simulink model "active_suspension_sim"  (Simulink 9.1)
settings: Solver=ode45  StartTime=0.0  StopTime=5  RelTol=1e-3
values from neighbouring files (symbols this model uses):
  A = [[0 1 0 0 0];[-(cw+cs)/mw -ds/mw cs/mw ds/mw -1/mw];[0 0 0 1 0];[cs/mc ds/mc -cs/mc -ds/mc 1/mc];[0 0 0 0 -1/tau]]    [active_suspension_ctrl_design.m]
  B1 = [B H]    [active_suspension_ctrl_design.m]
  C = [[-1 0 1 0 0];[cs/mc ds/mc -cs/mc -ds/mc 1/mc]]    [active_suspension_ctrl_design.m]
  C1 = eye(5)    [active_suspension_ctrl_design.m]
  D1 = zeros(5,2)    [active_suspension_ctrl_design.m]
  ds = 2200    [active_suspension_ctrl_design.m]
undefined symbols (not defined in the file or in its folder): K
libraries: simulink x3
settings Model: Creator=JonasMac  LastModifiedBy=joses
settings DataIOCC: LimitDataPoints=on  SignalLoggingSaveFormat=ModelDataLogs
settings OptimizationCC: BlockReduction=off  BooleanDataType=off
settings DebuggingCC: SaveWithParameterizedLinksMsg=none  SignalResolutionControl=TryResolveAllWithWarning  MultiTaskDSMMsg=warning  MultiTaskCondExecSysMsg=none
settings HardwareCC: TargetUnknown=on
settings GRTTargetCC: CombineOutputUpdateFcns=on  GRTInterface=off

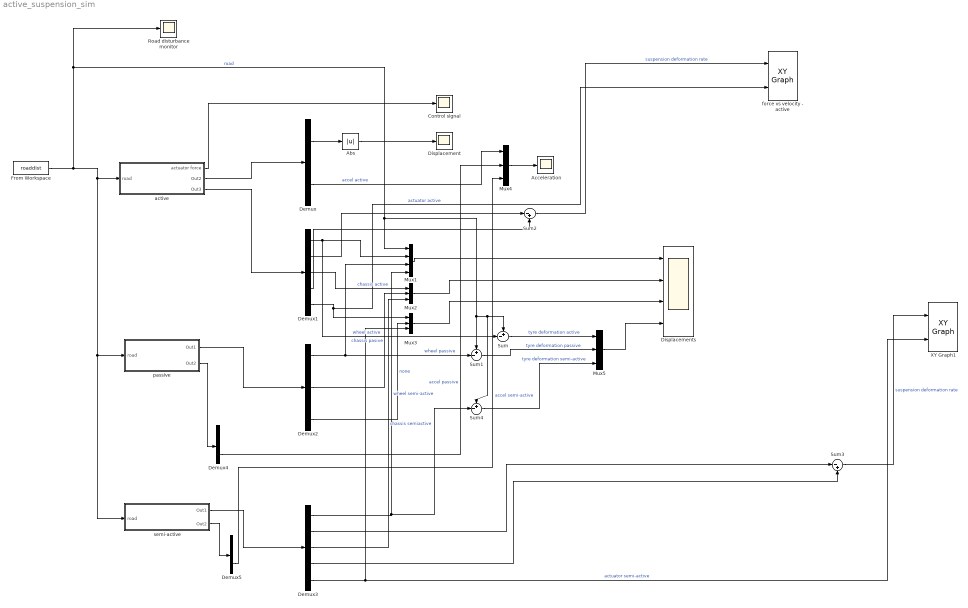
== system active_suspension_sim ==
  Abs : Abs
  Acceleration : Scope
  Control signal : Scope
  Demux : Demux  Outputs=2
  Demux1 : Demux  Outputs=5
  Demux2 : Demux  Outputs=5
  Demux3 : Demux  Outputs=5
  Demux4 : Demux  Outputs=2
  Demux5 : Demux  Outputs=2
  Displacement : Scope
  Displacements : Scope  NumInputPorts=4
  From Workspace : FromWorkspace  VariableName=roaddist  SampleTime=0
  Mux1 : Mux
  Mux{2..5} (4 alike) : Mux  Inputs=3
  Road disturbance monitor : Scope
  Sum : Sum  Inputs=+-|
  Sum1 : Sum  Inputs=+-|
  Sum2 : Sum  Inputs=|-+
  Sum3 : Sum  Inputs=|-+
  Sum4 : Sum  Inputs=+-|
  XY Graph1 : simulink/Sinks/XY Graph  xmin=-inf  xmax=inf  ymin=-inf  ymax=inf  st=.01
  active : Subsystem
  force vs velocity - active : simulink/Sinks/XY Graph  xmin=-inf  xmax=inf  ymin=-inf  ymax=inf  st=.01
  passive : Subsystem
  semi-active : Subsystem
  wires:
  Demux/1 -> Abs/1
  Abs/1 -> Displacement/1
  Mux1/1 -> Displacements/1
  Mux2/1 -> Displacements/2
  Mux3/1 -> Displacements/3
  Demux1/1 -> Sum/2, Mux1/2  "wheel active"
  Demux2/1 -> Sum1/2, Mux1/3  "wheel passive"
  Demux1/3 -> Mux2/1  "chassis active"
  Demux2/3 -> Mux2/2  "chassis pasive"
  Demux1/5 -> force vs velocity - active/2, Mux3/1  "actuator active"
  Demux2/5 -> Mux3/2  "none"
  Mux5/1 -> Displacements/4
  Sum/1 -> Mux5/1  "tyre deformation active"
  Sum1/1 -> Mux5/2  "tyre deformation passive"
  Demux1/2 -> Sum2/1
  Demux1/4 -> Sum2/2
  Sum2/1 -> force vs velocity - active/1  "suspension deformation rate"
  From Workspace/1 -> Road disturbance monitor/1, Sum1/1, Sum4/1, Sum/1, Mux1/1, semi-active/1(road), passive/1(road), active/1(road)  "road"
  active/1(actuator force) -> Control signal/1
  active/2(Out2) -> Demux/1
  active/3(Out3) -> Demux1/1
  passive/1(Out1) -> Demux2/1
  semi-active/1(Out1) -> Demux3/1
  Demux3/1 -> Sum4/2, Mux1/4  "wheel semi-active"
  Demux3/3 -> Mux2/3  "chassis semiactive"
  Demux3/5 -> XY Graph1/2, Mux3/3  "actuator semi-active"
  Sum3/1 -> XY Graph1/1  "suspension deformation rate"
  Demux3/4 -> Sum3/2
  Demux3/2 -> Sum3/1
  Sum4/1 -> Mux5/3  "tyre deformation semi-active"
  Mux4/1 -> Acceleration/1
  Demux/2 -> Mux4/1  "accel active"
  semi-active/2(Out2) -> Demux5/1
  Demux5/2 -> Mux4/3  "accel semi-active"
  passive/2(Out2) -> Demux4/1
  Demux4/2 -> Mux4/2  "accel passive"

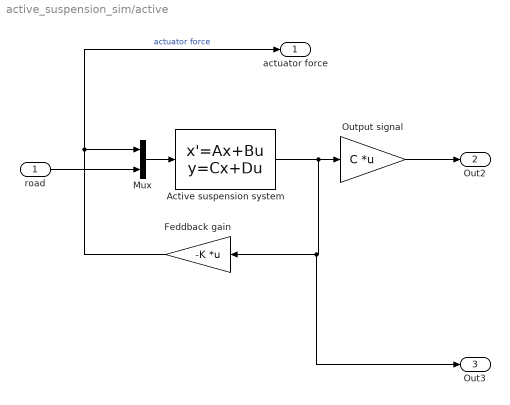
== system active_suspension_sim/active ==
  road : Inport
  Active suspension system : StateSpace  A=A  B=B1  C=C1  D=D1
  Feddback gain : Gain  Gain=-K  Multiplication=Matrix(K*u)
  Mux : Mux  Inputs=2
  Output signal : Gain  Gain=C  Multiplication=Matrix(K*u)
  actuator force : Outport
  Out2 : Outport  Port=2
  Out3 : Outport  Port=3
  wires:
  Active suspension system/1 -> Out3/1, Feddback gain/1, Output signal/1
  Feddback gain/1 -> actuator force/1, Mux/1  "actuator force"
  Mux/1 -> Active suspension system/1
  road/1 -> Mux/2
  Output signal/1 -> Out2/1

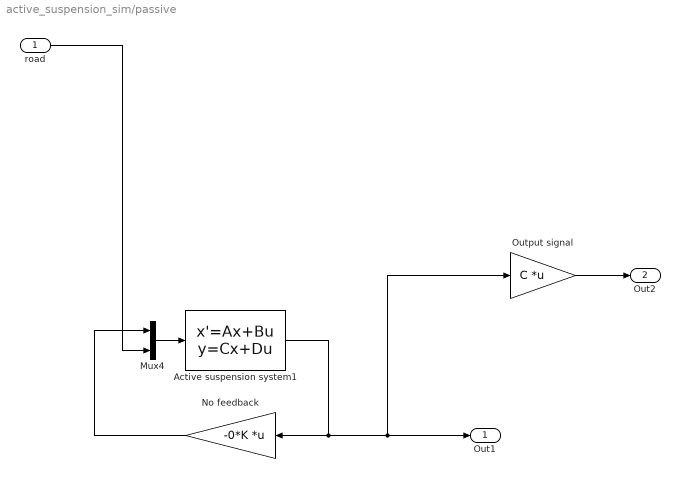
== system active_suspension_sim/passive ==
  road : Inport
  Active suspension system1 : StateSpace  A=A  B=B1  C=C1  D=D1
  Mux4 : Mux  Inputs=2
  No feedback : Gain  Gain=-0*K  Multiplication=Matrix(K*u)
  Output signal : Gain  Gain=C  Multiplication=Matrix(K*u)
  Out1 : Outport
  Out2 : Outport  Port=2
  wires:
  road/1 -> Mux4/2
  Active suspension system1/1 -> Output signal/1, Out1/1, No feedback/1
  Mux4/1 -> Active suspension system1/1
  No feedback/1 -> Mux4/1
  Output signal/1 -> Out2/1

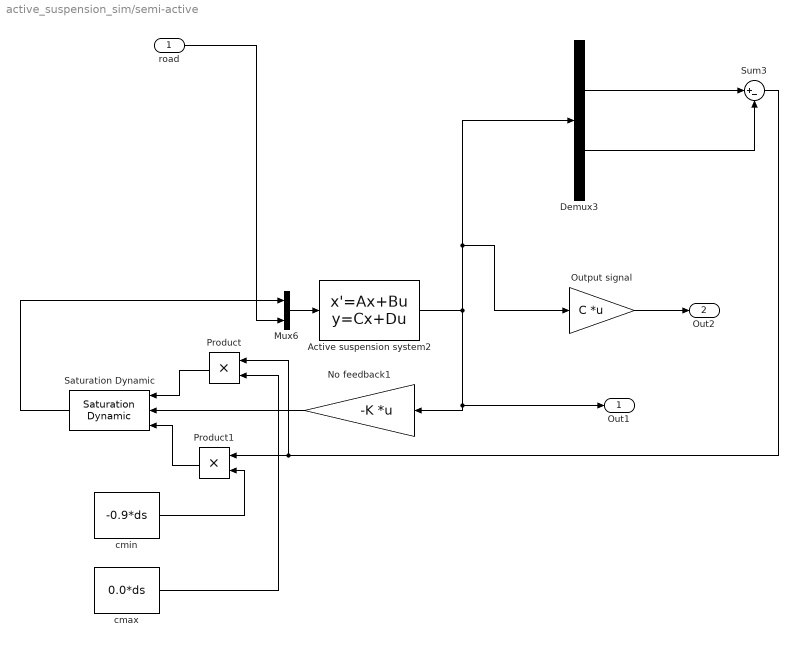
== system active_suspension_sim/semi-active ==
  road : Inport
  Active suspension system2 : StateSpace  A=A  B=B1  C=C1  D=D1
  Demux3 : Demux  Outputs=5
  Mux6 : Mux  Inputs=2
  No feedback1 : Gain  Gain=-K  Multiplication=Matrix(K*u)
  Output signal : Gain  Gain=C  Multiplication=Matrix(K*u)
  Product : Product
  Product1 : Product
  Saturation Dynamic : simulink/Discontinuities/Saturation Dynamic  OutMin=[]  OutMax=[]  OutDataTypeStr=Inherit: Same as second input  OutDataType=fixdt(1, 16)  OutScaling=2^-10  DoSatur=off
  Sum3 : Sum  Inputs=|+-
  cmax : Constant  Value=0.0*ds
  cmin : Constant  Value=-0.9*ds
  Out1 : Outport
  Out2 : Outport  Port=2
  wires:
  Active suspension system2/1 -> Output signal/1, Demux3/1, Out1/1, No feedback1/1
  Mux6/1 -> Active suspension system2/1
  road/1 -> Mux6/2
  Demux3/2 -> Sum3/1
  Demux3/4 -> Sum3/2
  No feedback1/1 -> Saturation Dynamic/2
  Saturation Dynamic/1 -> Mux6/1
  Product/1 -> Saturation Dynamic/1
  Product1/1 -> Saturation Dynamic/3
  cmin/1 -> Product1/2
  Sum3/1 -> Product/1, Product1/1
  cmax/1 -> Product/2
  Output signal/1 -> Out2/1
